simulink model "M11_sim"  (R2021b)
settings: Solver=VariableStepAuto  StartTime=0.0  StopTime=3  RelTol=1e-3
values from neighbouring files (symbols this model uses):
  K1 = wn^2    [M10.m]    (also in M11.m = wn * wn)
  K2 = 2*zeta*wn    [M10.m]    (also in M11.m = 2*zeta*wn - 1)
  wn = BW / (sqrt((1 - 2*zeta^2) + sqrt(4*zeta^4 - 4*zeta^2 +2)))    [M10.m]    (also in M11.m = pi/(tp * sqrt(1 - (zeta * zeta))))
  zeta = rzeta(4)    [M10.m]    (also in M11.m = 1 / sqrt(a * a + 1))
settings Model: Creator=Studenci  LastModifiedBy=Studenci

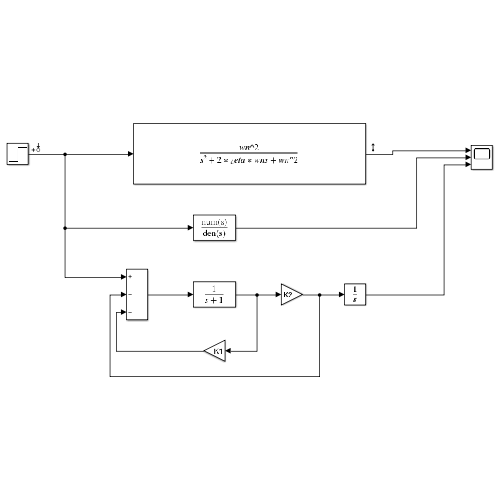
[thumbnail: Simulink's stored preview of the top-level diagram]
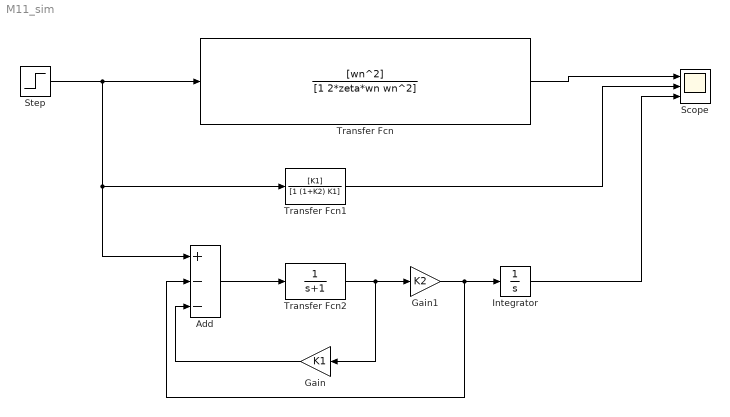
== system M11_sim ==
  Add : Sum  Inputs=+--
  Gain : Gain  Gain=K1
  Gain1 : Gain  Gain=K2
  Integrator : Integrator
  Scope : Scope  NumInputPorts=3
  Step : Step  SampleTime=0
  Transfer Fcn : TransferFcn  Numerator=[wn^2]  Denominator=[1 2*zeta*wn wn^2]
  Transfer Fcn1 : TransferFcn  Numerator=[K1]  Denominator=[1 (1+K2) K1]
  Transfer Fcn2 : TransferFcn  Denominator=[1 1]
  wires:
  Step/1 -> Transfer Fcn1/1, Add/1, Transfer Fcn/1
  Transfer Fcn/1 -> Scope/1
  Gain/1 -> Add/3
  Add/1 -> Transfer Fcn2/1
  Transfer Fcn2/1 -> Gain/1, Gain1/1
  Gain1/1 -> Add/2, Integrator/1
  Integrator/1 -> Scope/3
  Transfer Fcn1/1 -> Scope/2
